simulink model "dataSchemeSimulink"  (R2021a)
settings: Solver=FixedStepDiscrete  StartTime=0.0  StopTime=18  RelTol=1e-3
model workspace (MAT data in the model file):
  firstWarning = 0
  originalScenarioChecksum = '7BF13A567A736ECA8B90B8EA7CEEEB38'
values from neighbouring files (symbols this model uses):
  C = [ 1   0   0   0; 0   0   1   0]    [lpvGainScheduled.m]    (also in main.m = [1 0 0 0;0 1 0 0;0 0 1 0;0 0 0 1])
  Ts = 0.01    [lpvGainScheduled.m]    (also in main.m)
libraries: drivingscenarioandsensors x1
settings Model: PacingRate=0.710000  Creator=nicol  LastModifiedBy=nicol

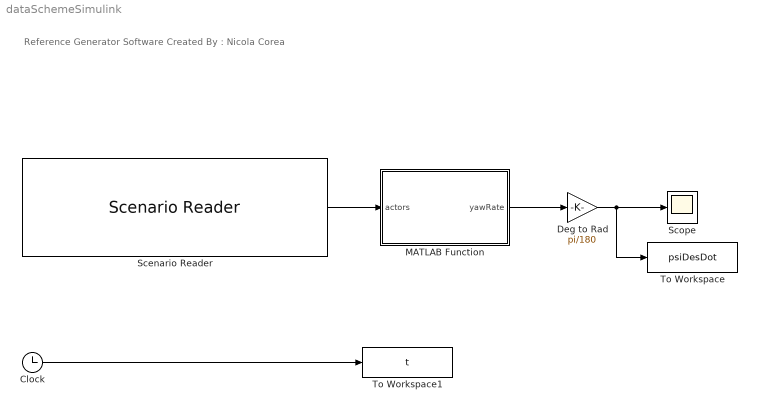
== system dataSchemeSimulink ==
  note: Reference Generator
      | Software Created By : Nicola Corea
  Clock : Clock
  Deg to Rad : Gain  Gain=pi/180
  MATLAB Function : MATLAB Function  TreatAsAtomicUnit=on
  Scenario Reader : drivingscenarioandsensors/Scenario Reader  ScenarioSource=From file  ScenarioFileName=C:\Users\nicol\Desktop\ProgettoFinale-NicolaCorea\Modulo2\DrivingScenarioLateral\obtainDataFromScenario.mat  ScenarioVariableName=scenario  OutputCoordinateSystem=Vehicle coordinates  EgoVehicleSource=Scenario  EgoVehicleActorID=1  OrientVehiclesOnRoad=off  OutputEgoVehiclePose=off  SampleTime=0.1  LaneBoundaryOutput=None  LaneBoundaryDistance=0:0.5:9.5  LaneBoundaryLocation=Center of lane markings  BusNameSource=Auto  BusName=BusActors  BusNumActorsSource=Scenario  BusNumActors=100  BusName2Source=Auto  BusName2=BusLaneBoundaries  BusNumLaneBoundariesSource=Scenario  BusNumLaneBoundaries=10  BusName3Source=Auto  BusName3=BusEgoActor  ShowCoordinateLabels=on  SimulateUsing=Interpreted execution
  Scope : Scope
  To Workspace : ToWorkspace  VariableName=psiDesDot  SampleTime=Ts
      settings: Save2DSignal=2-D array (concatenate along first dimension)
  To Workspace1 : ToWorkspace  VariableName=t  SampleTime=Ts
      settings: Save2DSignal=2-D array (concatenate along first dimension)
  wires:
  Scenario Reader/1 -> MATLAB Function/1(actors)
  MATLAB Function/1(yawRate) -> Deg to Rad/1
  Deg to Rad/1 -> To Workspace/1, Scope/1
  Clock/1 -> To Workspace1/1

== matlab function dataSchemeSimulink/MATLAB Function ==
  data: actors input; yawRate output
function yawRate  = getDesiredOrientation(actors)
% Selecting Actor
actor   = actors.Actors(1);
% Obtaining Desired Yaw Rate
aVel    = actor.AngularVelocity;
yawRate = aVel(3);
end
